simulink library "rampSaturatedXYZT"  (R2020a)
settings: Solver=VariableStepAuto  StartTime=0.0  StopTime=10.0  RelTol=1e-3
undefined symbols (not defined in the file): env, flowSpeedOpenLoop, rampSlope
libraries: simulink x1
settings Model: Creator=jcreed2  LastModifiedBy=jcreed2

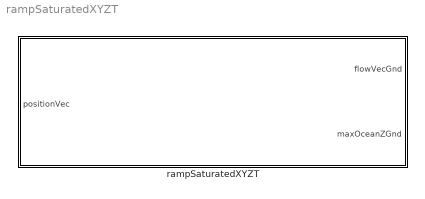
== system rampSaturatedXYZT ==
  rampSaturatedXYZT : Subsystem  mask{constXYZT=env.water}
      mask prompts: constXYZT "env.constXYZT Object"

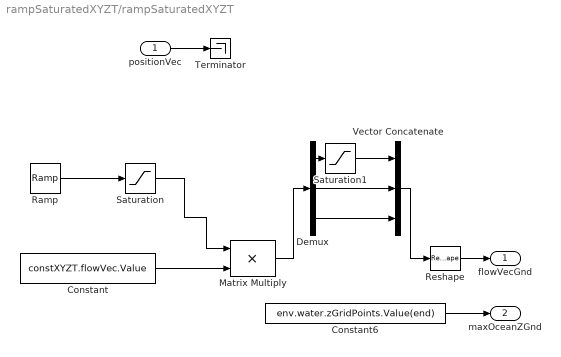
== system rampSaturatedXYZT/rampSaturatedXYZT ==
  positionVec : Inport
  Constant : Constant  Value=constXYZT.flowVec.Value
  Constant6 : Constant  Value=env.water.zGridPoints.Value(end)
  Demux : Demux  Outputs=3
  Matrix Multiply : Product
  Ramp : simulink/Sources/Ramp  slope=rampSlope  start=fltCtrl.startControl.Value  InitialOutput=0
  Reshape : Reshape  OutputDimensionality=Column vector (2-D)
  Saturation : Saturate  UpperLimit=1  LowerLimit=0
  Saturation1 : Saturate  UpperLimit=flowSpeedOpenLoop  LowerLimit=-inf
  Terminator : Terminator
  Vector Concatenate : Concatenate  NumInputs=3
  flowVecGnd : Outport  VectorParamsAs1DForOutWhenUnconnected=off
  maxOceanZGnd : Outport  Port=2  VectorParamsAs1DForOutWhenUnconnected=off
  wires:
  Constant/1 -> Matrix Multiply/2
  positionVec/1 -> Terminator/1
  Constant6/1 -> maxOceanZGnd/1
  Reshape/1 -> flowVecGnd/1
  Ramp/1 -> Saturation/1
  Saturation/1 -> Matrix Multiply/1
  Matrix Multiply/1 -> Demux/1
  Saturation1/1 -> Vector Concatenate/1
  Demux/1 -> Saturation1/1
  Demux/3 -> Vector Concatenate/3
  Demux/2 -> Vector Concatenate/2
  Vector Concatenate/1 -> Reshape/1
